simulink model "Eom_VarLocalLevelQuat"  (R2016b)
settings: Solver=VariableStepAuto  StartTime=0.0  StopTime=10.0  RelTol=1e-3
undefined symbols (not defined in the file or in its folder): Sim
libraries: OpenFlightUtilLib x8, SimCoreLib x1
settings Model: Creator=rega0051  LastModifiedBy=rega0051
settings DataIOCC: SaveOutput=off  SignalLogging=off  DSMLogging=off  SaveTime=off

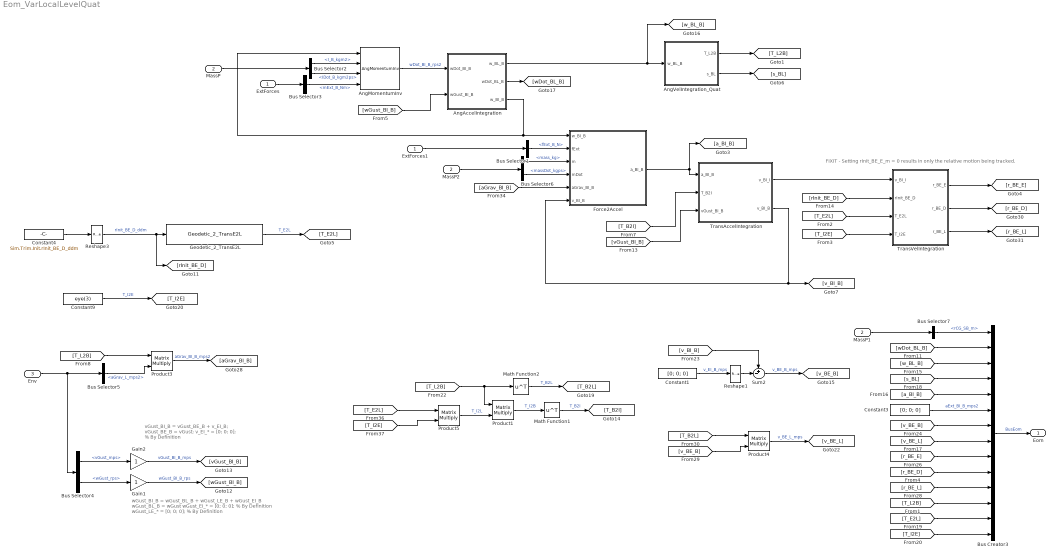
== system Eom_VarLocalLevelQuat ==
  note: FIXIT - Setting rInit_BE_E_m = 0 results in only the relative motion being tracked.
  note: vGust_BI_B = vGust_BE_B + v_EI_B;
      | vGust_BE_B = vGust;
      | v_EI_* = [0; 0; 0]; % By Definition
  note: wGust_BI_B = wGust_BL_B + wGust_LE_B + wGust_EI_B
      | wGust_BL_B = wGust
      | wGust_EI_* = [0; 0; 0]; % By Definition
      | wGust_LE_* = [0; 0; 0]; % By Definition
  ExtForces : Inport  OutDataTypeStr=Bus: BusExtForce
      settings: AttributesFormatString=%<OutDataTypeStr>
  MassP : Inport  Port=2  OutDataTypeStr=Bus: BusMassP
      settings: AttributesFormatString=%<OutDataTypeStr>
  Env : Inport  Port=3  OutDataTypeStr=Bus: BusEnv
      settings: AttributesFormatString=%<OutDataTypeStr>
  AngAccelIntegration : Subsystem
  AngMomentumInv : OpenFlightUtilLib/Kinematics and Dynamics/AngMomentumInv
  AngVelIntegration_Quat : Subsystem
  Bus Selector1 : BusSelector  OutputSignals=fExt_B_N
  Bus Selector2 : BusSelector  OutputSignals=I_B_kgm2,IDot_B_kgm2ps
  Bus Selector3 : BusSelector  OutputSignals=mExt_B_Nm
  Bus Selector4 : BusSelector  OutputSignals=BusAtmos.vGust_mps,BusAtmos.wGust_rps
  Bus Selector5 : BusSelector  OutputSignals=BusGrav.aGrav_L_mps2
  Bus Selector6 : BusSelector  OutputSignals=mass_kg,massDot_kgps
  Bus Selector7 : BusSelector  OutputSignals=rCG_SB_m
  Bus Creator3 : BusCreator  Inputs=14  OutDataTypeStr=Bus: BusEom  NonVirtualBus=on
      settings: AttributesFormatString=%<OutDataTypeStr>  InheritFromInputs=off
  Constant1 : Constant  Value=[0; 0; 0]
      settings: AttributesFormatString=%<Value>
  Constant3 : Constant  Value=[0; 0; 0]
      settings: AttributesFormatString=%<Value>
  Constant4 : Constant  Value=Sim.Trim.Init.rInit_BE_D_ddm
      settings: AttributesFormatString=%<Value>
  Constant9 : Constant  Value=eye(3)
      settings: AttributesFormatString=%<Value>
  Force2Accel : Subsystem
  Gain1 : Gain
  Gain2 : Gain
  Geodetic_2_TransE2L : OpenFlightUtilLib/Transformations/Geodetic_2_TransE2L
  ExtForces1 : InportShadow  OutDataTypeStr=Bus: BusExtForce
      settings: AttributesFormatString=%<OutDataTypeStr>
  MassP1 : InportShadow  Port=2  OutDataTypeStr=Bus: BusMassP
      settings: AttributesFormatString=%<OutDataTypeStr>
  MassP2 : InportShadow  Port=2  OutDataTypeStr=Bus: BusMassP
      settings: AttributesFormatString=%<OutDataTypeStr>
  Math Function1 : Math  Operator=transpose  SaturateOnIntegerOverflow=on
  Math Function2 : Math  Operator=transpose  SaturateOnIntegerOverflow=on
  Product{1,3..5} (4 alike) : Product  Inputs=**  Multiplication=Matrix(*)  RndMeth=Zero
  Reshape1 : Reshape  OutputDimensionality=Column vector (2-D)  OutputDimensions=[3,1]
  Reshape3 : Reshape  OutputDimensionality=Column vector (2-D)  OutputDimensions=[3,1]
  Sum2 : Sum  Inputs=+-|
  TransAccelIntegration : Subsystem
  TransVelIntegration : Subsystem
  Eom : Outport  OutDataTypeStr=Bus: BusEom
      settings: AttributesFormatString=%<OutDataTypeStr>
  wires:
  Reshape3/1 -> Geodetic_2_TransE2L/1, [rInit_BE_D]  "rInit_BE_D_ddm"
  Math Function1/1 -> [T_B2I]  "T_B2I"
  Product1/1 -> Math Function1/1  "T_I2B"
  [T_B2I] -> TransAccelIntegration/2(T_B2I)
  TransVelIntegration/1(r_BE_E) -> [r_BE_E]
  TransAccelIntegration/1(v_BI_I) -> TransVelIntegration/1(v_BI_I)
  Bus Selector6/2 -> Force2Accel/4(mDot)  "<massDot_kgps>"
  Bus Selector6/1 -> Force2Accel/3(m)  "<mass_kg>"
  Product3/1 -> [aGrav_BI_B]  "aGrav_BI_B_mps2"
  AngVelIntegration_Quat/1(T_L2B) -> [T_L2B]
  Bus Selector1/1 -> Force2Accel/2(fExt)  "<fExt_B_N>"
  Bus Creator3/1 -> Eom/1  "BusEom"
  [T_L2B] -> Bus Creator3/12
  ExtForces1/1 -> Bus Selector1/1
  Bus Selector5/1 -> Product3/2  "<aGrav_L_mps2>"
  [T_L2B] -> Product3/1
  AngVelIntegration_Quat/2(s_BL) -> [s_BL]
  Force2Accel/1(a_BI_B) -> [a_BI_B], TransAccelIntegration/1(a_BI_B)
  AngMomentumInv/1 -> AngAccelIntegration/1(wDot_BI_B)  "wDot_BI_B_rps2"
  Bus Selector2/1 -> AngMomentumInv/2  "<I_B_kgm2>"
  Bus Selector2/2 -> AngMomentumInv/3  "<IDot_B_kgm2ps>"
  Bus Selector3/1 -> AngMomentumInv/4  "<mExt_B_Nm>"
  [s_BL] -> Bus Creator3/4
  [a_BI_B] -> Bus Creator3/5
  [r_BE_D] -> Bus Creator3/10
  [w_BL_B] -> Bus Creator3/3
  [wDot_BL_B] -> Bus Creator3/2
  [v_BE_L] -> Bus Creator3/8
  AngAccelIntegration/1(w_BL_B) -> [w_BL_B], AngVelIntegration_Quat/1(w_BL_B)
  [T_E2L] -> Bus Creator3/13
  [T_I2E] -> Bus Creator3/14
  Geodetic_2_TransE2L/1 -> [T_E2L]  "T_E2L"
  Constant9/1 -> [T_I2E]  "T_I2E"
  [T_L2B] -> Product1/1, Math Function2/1
  Product4/1 -> [v_BE_L]  "v_BE_L_mps"
  [r_BE_L] -> Bus Creator3/11
  [v_BE_B] -> Product4/2
  [T_B2L] -> Product4/1
  Product5/1 -> Product1/2  "T_I2L"
  Bus Selector4/1 -> Gain2/1  "<vGust_mps>"
  [aGrav_BI_B] -> Force2Accel/5(aGrav_BI_B)
  AngAccelIntegration/2(wDot_BL_B) -> [wDot_BL_B]
  TransVelIntegration/2(r_BE_D) -> [r_BE_D]
  TransVelIntegration/3(r_BE_L) -> [r_BE_L]
  [rInit_BE_D] -> TransVelIntegration/2(rInit_BE_D)
  [T_I2E] -> Product5/2
  [T_E2L] -> Product5/1
  MassP/1 -> Bus Selector2/1
  Bus Selector7/1 -> Bus Creator3/1  "<rCG_SB_m>"
  [wGust_BI_B] -> AngAccelIntegration/2(wGust_BI_B)
  Env/1 -> Bus Selector4/1, Bus Selector5/1
  Bus Selector4/2 -> Gain1/1  "<wGust_rps>"
  Gain2/1 -> [vGust_BI_B]  "vGust_BI_B_mps"
  Gain1/1 -> [wGust_BI_B]  "wGust_BI_B_rps"
  [vGust_BI_B] -> TransAccelIntegration/3(vGust_BI_B)
  [v_BE_B] -> Bus Creator3/7
  [r_BE_E] -> Bus Creator3/9
  [T_E2L] -> TransVelIntegration/3(T_E2L)
  Sum2/1 -> [v_BE_B]  "v_BE_B_mps"
  Constant1/1 -> Reshape1/1  "v_EI_B_mps"
  [v_BI_B] -> Sum2/1
  Math Function2/1 -> [T_B2L]  "T_B2L"
  Reshape1/1 -> Sum2/2
  AngAccelIntegration/3(w_BI_B) -> Force2Accel/1(w_BI_B), AngMomentumInv/1
  TransAccelIntegration/2(v_BI_B) -> [v_BI_B], Force2Accel/6(v_BI_B)
  Constant3/1 -> Bus Creator3/6  "aExt_BI_B_mps2"
  Constant4/1 -> Reshape3/1
  [T_I2E] -> TransVelIntegration/4(T_I2E)
  MassP1/1 -> Bus Selector7/1
  ExtForces/1 -> Bus Selector3/1
  MassP2/1 -> Bus Selector6/1

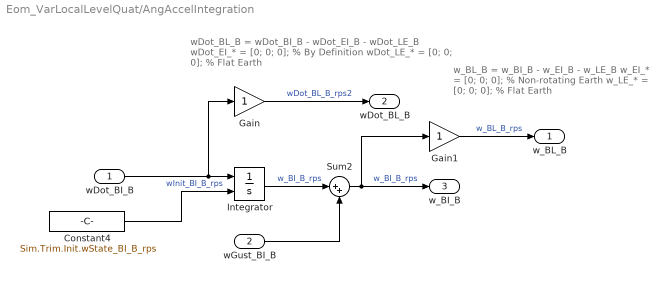
== system Eom_VarLocalLevelQuat/AngAccelIntegration ==
  note: w_BL_B = w_BI_B - w_EI_B - w_LE_B
      | w_EI_* = [0; 0; 0]; % Non-rotating Earth
      | w_LE_* = [0; 0; 0]; % Flat Earth
  note: wDot_BL_B = wDot_BI_B - wDot_EI_B - wDot_LE_B
      | wDot_EI_* = [0; 0; 0]; % By Definition
      | wDot_LE_* = [0; 0; 0]; % Flat Earth
  wDot_BI_B : Inport
  wGust_BI_B : Inport  Port=2
  Constant4 : Constant  Value=Sim.Trim.Init.wState_BI_B_rps
      settings: AttributesFormatString=%<Value>
  Gain : Gain
  Gain1 : Gain
  Integrator : Integrator  InitialConditionSource=external  ContinuousStateAttributes='wState_BI_B_rps'
      settings: AttributesFormatString=State: %<ContinuousStateAttributes>
  Sum2 : Sum  Inputs=|++  SaturateOnIntegerOverflow=on
  w_BL_B : Outport
  wDot_BL_B : Outport  Port=2
  w_BI_B : Outport  Port=3
  wires:
  Constant4/1 -> Integrator/2  "wInit_BI_B_rps"
  wGust_BI_B/1 -> Sum2/2
  Gain/1 -> wDot_BL_B/1  "wDot_BL_B_rps2"
  Gain1/1 -> w_BL_B/1  "w_BL_B_rps"
  wDot_BI_B/1 -> Gain/1, Integrator/1
  Integrator/1 -> Sum2/1  "w_BI_B_rps"
  Sum2/1 -> w_BI_B/1, Gain1/1  "w_BI_B_rps"

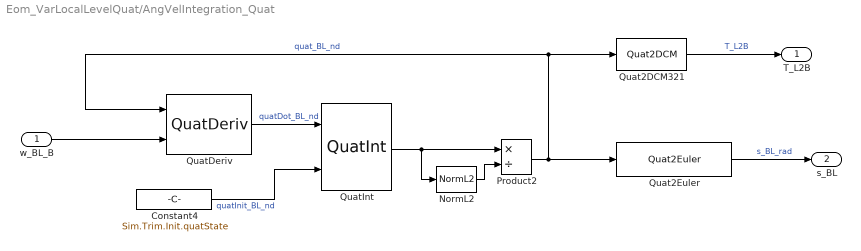
== system Eom_VarLocalLevelQuat/AngVelIntegration_Quat ==
  w_BL_B : Inport
  Constant4 : Constant  Value=Sim.Trim.Init.quatState
      settings: AttributesFormatString=%<Value>
  NormL2 : OpenFlightUtilLib/Math/NormL2
  Product2 : Product  Inputs=*/  RndMeth=Zero
  Quat2DCM321 : OpenFlightUtilLib/Transformations/Quat2DCM
  Quat2Euler : OpenFlightUtilLib/Transformations/Quat2Euler
  QuatDeriv : OpenFlightUtilLib/Transformations/QuatDeriv
  QuatInt : OpenFlightUtilLib/Transformations/QuatInt
  T_L2B : Outport
  s_BL : Outport  Port=2
  wires:
  Quat2Euler/1 -> s_BL/1  "s_BL_rad"
  Quat2DCM321/1 -> T_L2B/1  "T_L2B"
  NormL2/1 -> Product2/2
  QuatDeriv/1 -> QuatInt/1  "quatDot_BL_nd"
  QuatInt/1 -> Product2/1, NormL2/1
  Product2/1 -> Quat2Euler/1, Quat2DCM321/1, QuatDeriv/1  "quat_BL_nd"
  Constant4/1 -> QuatInt/2  "quatInit_BL_nd"
  w_BL_B/1 -> QuatDeriv/2

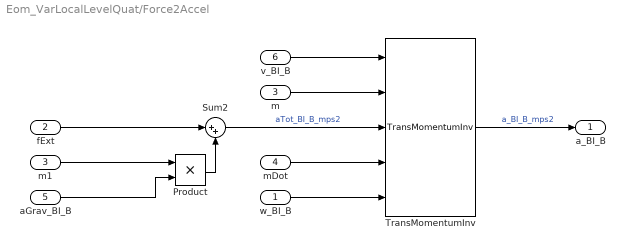
== system Eom_VarLocalLevelQuat/Force2Accel ==
  w_BI_B : Inport
  fExt : Inport  Port=2
  m : Inport  Port=3
  mDot : Inport  Port=4
  aGrav_BI_B : Inport  Port=5
  v_BI_B : Inport  Port=6
  Product : Product
  Sum2 : Sum  Inputs=|++  SaturateOnIntegerOverflow=on
  TransMomentumInv : OpenFlightUtilLib/Kinematics and Dynamics/TransMomentumInv
  m1 : InportShadow  Port=3
  a_BI_B : Outport
  wires:
  Sum2/1 -> TransMomentumInv/3  "aTot_BI_B_mps2"
  Product/1 -> Sum2/2
  m1/1 -> Product/1
  fExt/1 -> Sum2/1
  v_BI_B/1 -> TransMomentumInv/1
  w_BI_B/1 -> TransMomentumInv/5
  mDot/1 -> TransMomentumInv/4
  m/1 -> TransMomentumInv/2
  aGrav_BI_B/1 -> Product/2
  TransMomentumInv/1 -> a_BI_B/1  "a_BI_B_mps2"

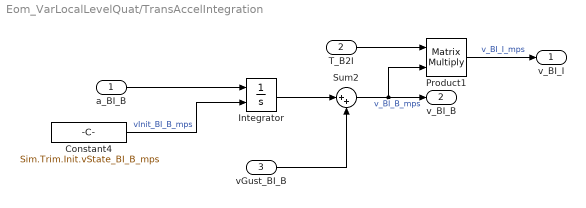
== system Eom_VarLocalLevelQuat/TransAccelIntegration ==
  a_BI_B : Inport
  T_B2I : Inport  Port=2
  vGust_BI_B : Inport  Port=3
  Constant4 : Constant  Value=Sim.Trim.Init.vState_BI_B_mps
      settings: AttributesFormatString=%<Value>
  Integrator : Integrator  InitialConditionSource=external  ContinuousStateAttributes='vState_BI_B_mps'
      settings: AttributesFormatString=State: %<ContinuousStateAttributes>
  Product1 : Product  Inputs=**  Multiplication=Matrix(*)  RndMeth=Zero
  Sum2 : Sum  Inputs=|++  SaturateOnIntegerOverflow=on
  v_BI_I : Outport
  v_BI_B : Outport  Port=2
  wires:
  Integrator/1 -> Sum2/1
  vGust_BI_B/1 -> Sum2/2
  Sum2/1 -> Product1/2, v_BI_B/1  "v_BI_B_mps"
  a_BI_B/1 -> Integrator/1
  T_B2I/1 -> Product1/1
  Product1/1 -> v_BI_I/1  "v_BI_I_mps"
  Constant4/1 -> Integrator/2  "vInit_BI_B_mps"

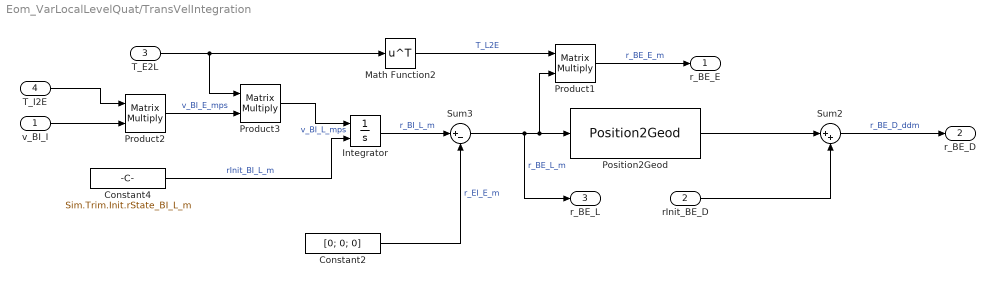
== system Eom_VarLocalLevelQuat/TransVelIntegration ==
  v_BI_I : Inport
  rInit_BE_D : Inport  Port=2
  T_E2L : Inport  Port=3
  T_I2E : Inport  Port=4
  Constant2 : Constant  Value=[0; 0; 0]
      settings: AttributesFormatString=%<Value>
  Constant4 : Constant  Value=Sim.Trim.Init.rState_BI_L_m
      settings: AttributesFormatString=%<Value>
  Integrator : Integrator  InitialConditionSource=external  ContinuousStateAttributes='rState_BI_L_m'
      settings: AttributesFormatString=State: %<ContinuousStateAttributes>
  Math Function2 : Math  Operator=transpose  SaturateOnIntegerOverflow=on
  Position2Geod : SimCoreLib/Position2Geod
  Product1 : Product  Inputs=**  Multiplication=Matrix(*)  RndMeth=Zero
  Product2 : Product  Inputs=**  Multiplication=Matrix(*)  RndMeth=Zero
  Product3 : Product  Inputs=**  Multiplication=Matrix(*)  RndMeth=Zero
  Sum2 : Sum  Inputs=|++
  Sum3 : Sum  Inputs=|+-
  r_BE_E : Outport
  r_BE_D : Outport  Port=2
  r_BE_L : Outport  Port=3
  wires:
  Product1/1 -> r_BE_E/1  "r_BE_E_m"
  Math Function2/1 -> Product1/1  "T_L2E"
  Product3/1 -> Integrator/1  "v_BI_L_mps"
  Product2/1 -> Product3/2  "v_BI_E_mps"
  T_I2E/1 -> Product2/1
  Constant4/1 -> Integrator/2  "rInit_BI_L_m"
  Constant2/1 -> Sum3/2  "r_EI_E_m"
  Sum3/1 -> Position2Geod/1, Product1/2, r_BE_L/1  "r_BE_L_m"
  rInit_BE_D/1 -> Sum2/2
  Sum2/1 -> r_BE_D/1  "r_BE_D_ddm"
  T_E2L/1 -> Product3/1, Math Function2/1
  Position2Geod/1 -> Sum2/1
  Integrator/1 -> Sum3/1  "r_BI_L_m"
  v_BI_I/1 -> Product2/2
